simulink model "Suspension_model"  (R2023a)
settings: Solver=ode1  StartTime=0.0  StopTime=10  FixedStep=0.001  RelTol=1e-3
values from neighbouring files (symbols this model uses):
  A = [ 0 1 0 -1 ... (first row only)    [FitnessFunc.m]
  B = [0  0 ... (first row only)    [FitnessFunc.m]
  C = [ 1 0 0 0 ... (first row only)    [FitnessFunc.m]
  D = [0 0 ... (first row only)    [FitnessFunc.m]
  k = lqr(A, B(:, 2), Q, R)    [FitnessFunc.m]
undefined symbols (not defined in the file or in its folder): K
settings Model: Creator=ku53058  LastModifiedBy=sevva
settings SolverCC: AlgebraicLoopSolver=TrustRegion
settings DataIOCC: ReturnWorkspaceOutputs=off
settings OptimizationCC: LifeSpan=inf
settings DebuggingCC: UnconnectedInputMsg=warning  UnconnectedOutputMsg=warning  UnconnectedLineMsg=warning  ArithmeticOperatorsInVariantConditions=warning
settings ModelReferenceCC: EnableRefExpFcnMdlSchedulingChecks=on
settings SFSimCC: SimUseLocalCustomCode=off  CustomCodeUndefinedFunction=UseInterfaceOnly
settings RTWCC: RTWUseLocalCustomCode=off
settings CodeAppCC: StateflowObjectComments=on

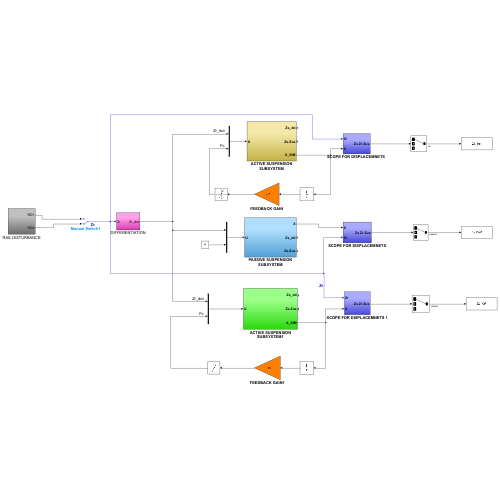
[thumbnail: Simulink's stored preview of the top-level diagram]
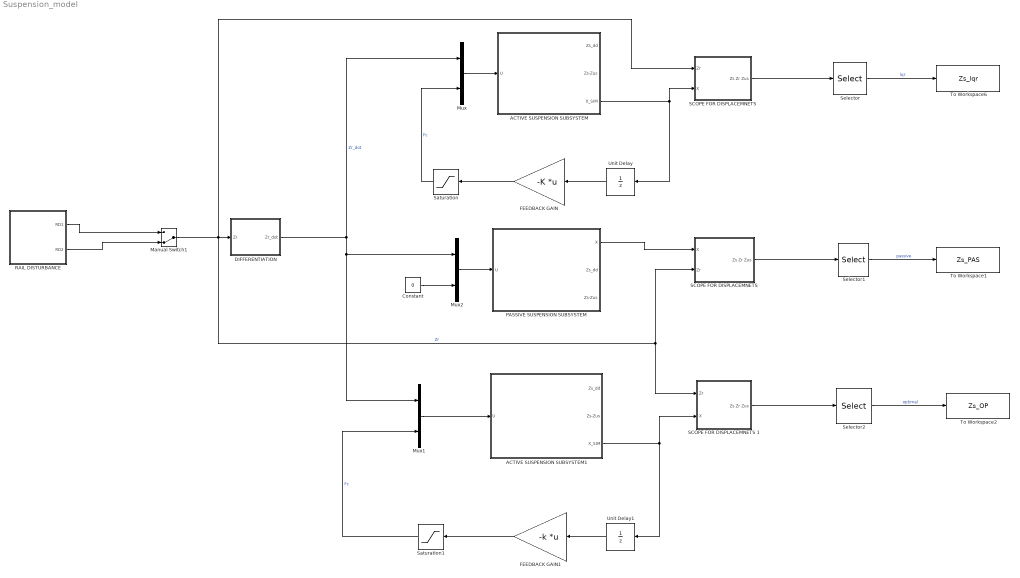
== system Suspension_model ==
  ACTIVE SUSPENSION SUBSYSTEM : Subsystem
  ACTIVE SUSPENSION SUBSYSTEM1 : Subsystem
  Constant : Constant  Value=0
  DIFFERENTIATION : Subsystem
  FEEDBACK GAIN : Gain  Gain=-K  Multiplication=Matrix(K*u)
  FEEDBACK GAIN1 : Gain  Gain=-k  Multiplication=Matrix(K*u)
  Manual Switch1 : ManualSwitch  CurrentSetting=0
  Mux : Mux  Inputs=2
  Mux1 : Mux  Inputs=2
  Mux2 : Mux  Inputs=2
  PASSIVE SUSPENSION SUBSYSTEM : Subsystem
  RAIL DISTURBANCE : Subsystem
  SCOPE FOR DISPLACEMNETS : Subsystem
  "SCOPE FOR DISPLACEMNETS " : Subsystem
  SCOPE FOR DISPLACEMNETS 1 : Subsystem
  Saturation : Saturate  UpperLimit=46730  LowerLimit=-46730
  Saturation1 : Saturate  UpperLimit=46730  LowerLimit=-46730
  Selector : Selector  InputPortWidth=3  IndexOptions=Index vector (dialog)  Indices=[1]  OutputSizes=1
  Selector1 : Selector  InputPortWidth=3  IndexOptions=Index vector (dialog)  Indices=[1]  OutputSizes=1
  Selector2 : Selector  InputPortWidth=3  IndexOptions=Index vector (dialog)  Indices=[1]  OutputSizes=1
  To Workspace1 : ToWorkspace  VariableName=Zs_PAS  SaveFormat=Timeseries  SampleTime=-1
  To Workspace2 : ToWorkspace  VariableName=Zs_OP  SaveFormat=Timeseries  SampleTime=-1
  To Workspace6 : ToWorkspace  VariableName=Zs_lqr  SaveFormat=Timeseries  SampleTime=-1
  Unit Delay : UnitDelay  SampleTime=-1  HasFrameUpgradeWarning=on
  Unit Delay1 : UnitDelay  SampleTime=-1  HasFrameUpgradeWarning=on
  wires:
  FEEDBACK GAIN/1 -> Saturation/1
  Constant/1 -> Mux2/2
  Unit Delay/1 -> FEEDBACK GAIN/1
  Saturation/1 -> Mux/2  "Fc"
  Mux/1 -> ACTIVE SUSPENSION SUBSYSTEM/1(U)
  ACTIVE SUSPENSION SUBSYSTEM/3(X_SIM) -> "SCOPE FOR DISPLACEMNETS "/2(X), Unit Delay/1
  "SCOPE FOR DISPLACEMNETS "/1(Zs Zr Zus) -> Selector/1
  Mux2/1 -> PASSIVE SUSPENSION SUBSYSTEM/1(U)
  PASSIVE SUSPENSION SUBSYSTEM/1(X) -> SCOPE FOR DISPLACEMNETS/1(X)
  SCOPE FOR DISPLACEMNETS/1(Zs Zr Zus) -> Selector1/1
  RAIL DISTURBANCE/1(RD1) -> Manual Switch1/1
  RAIL DISTURBANCE/2(RD2) -> Manual Switch1/2
  Selector/1 -> To Workspace6/1  "lqr"
  SCOPE FOR DISPLACEMNETS 1/1(Zs Zr Zus) -> Selector2/1
  Mux1/1 -> ACTIVE SUSPENSION SUBSYSTEM1/1(U)
  FEEDBACK GAIN1/1 -> Saturation1/1
  Unit Delay1/1 -> FEEDBACK GAIN1/1
  DIFFERENTIATION/1(Zr_dot) -> Mux/1, Mux1/1, Mux2/1  "Zr_dot"
  Saturation1/1 -> Mux1/2  "Fc"
  Manual Switch1/1 -> SCOPE FOR DISPLACEMNETS 1/1(Zr), SCOPE FOR DISPLACEMNETS/2(Zr), "SCOPE FOR DISPLACEMNETS "/1(Zr), DIFFERENTIATION/1(Zr)  "Zr"
  ACTIVE SUSPENSION SUBSYSTEM1/3(X_SIM) -> Unit Delay1/1, SCOPE FOR DISPLACEMNETS 1/2(X)
  Selector2/1 -> To Workspace2/1  "optimal"
  Selector1/1 -> To Workspace1/1  "passive"

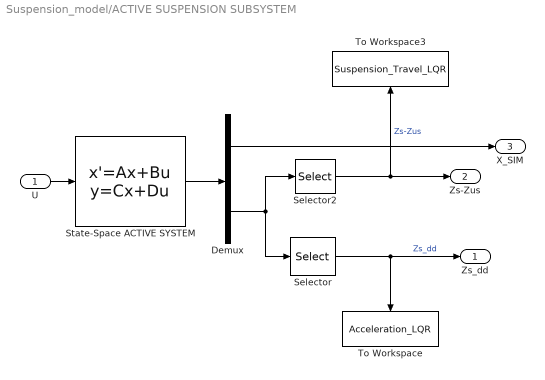
== system Suspension_model/ACTIVE SUSPENSION SUBSYSTEM ==
  U : Inport
  Demux : Demux  Outputs=[4 2]
  Selector : Selector  InputPortWidth=2  IndexOptions=Index vector (dialog)  Indices=[2]  OutputSizes=1
  Selector2 : Selector  InputPortWidth=2  IndexOptions=Index vector (dialog)  Indices=[1]  OutputSizes=1
  State-Space ACTIVE SYSTEM : StateSpace  A=A  B=B  C=cat(1,eye(4), C)  D=D  InitialCondition=0
  To Workspace : ToWorkspace  VariableName=Acceleration_LQR  SaveFormat=Timeseries  SampleTime=-1
  To Workspace3 : ToWorkspace  VariableName=Suspension_Travel_LQR  SaveFormat=Timeseries  SampleTime=-1
  Zs_dd : Outport
  Zs-Zus : Outport  Port=2
  X_SIM : Outport  Port=3
  wires:
  Demux/1 -> X_SIM/1
  State-Space ACTIVE SYSTEM/1 -> Demux/1
  Demux/2 -> Selector2/1, Selector/1
  Selector/1 -> Zs_dd/1, To Workspace/1  "Zs_dd"
  Selector2/1 -> Zs-Zus/1, To Workspace3/1  "Zs-Zus"
  U/1 -> State-Space ACTIVE SYSTEM/1

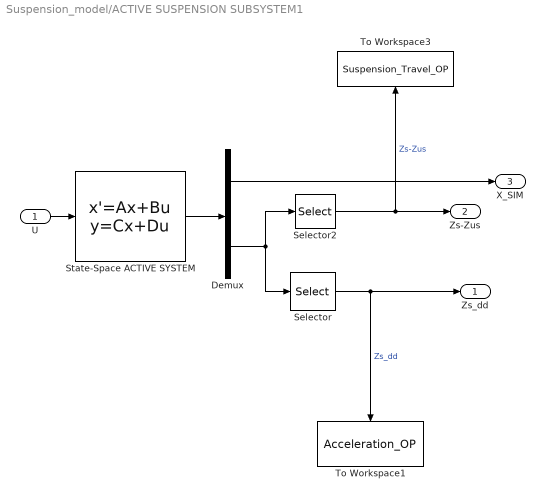
== system Suspension_model/ACTIVE SUSPENSION SUBSYSTEM1 ==
  U : Inport
  Demux : Demux  Outputs=[4 2]
  Selector : Selector  InputPortWidth=2  IndexOptions=Index vector (dialog)  Indices=[2]  OutputSizes=1
  Selector2 : Selector  InputPortWidth=2  IndexOptions=Index vector (dialog)  Indices=[1]  OutputSizes=1
  State-Space ACTIVE SYSTEM : StateSpace  A=A  B=B  C=cat(1,eye(4), C)  D=D  InitialCondition=0
  To Workspace1 : ToWorkspace  VariableName=Acceleration_OP  SaveFormat=Timeseries  SampleTime=-1
  To Workspace3 : ToWorkspace  VariableName=Suspension_Travel_OP  SaveFormat=Timeseries  SampleTime=-1
  Zs_dd : Outport
  Zs-Zus : Outport  Port=2
  X_SIM : Outport  Port=3
  wires:
  Demux/1 -> X_SIM/1
  State-Space ACTIVE SYSTEM/1 -> Demux/1
  Demux/2 -> Selector2/1, Selector/1
  Selector/1 -> To Workspace1/1, Zs_dd/1  "Zs_dd"
  Selector2/1 -> Zs-Zus/1, To Workspace3/1  "Zs-Zus"
  U/1 -> State-Space ACTIVE SYSTEM/1

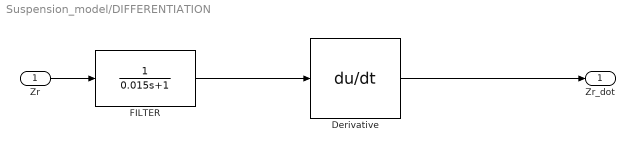
== system Suspension_model/DIFFERENTIATION ==
  Zr : Inport
  Derivative : Derivative
  FILTER : TransferFcn  Denominator=[0.015 1]
  Zr_dot : Outport
  wires:
  FILTER/1 -> Derivative/1
  Derivative/1 -> Zr_dot/1
  Zr/1 -> FILTER/1

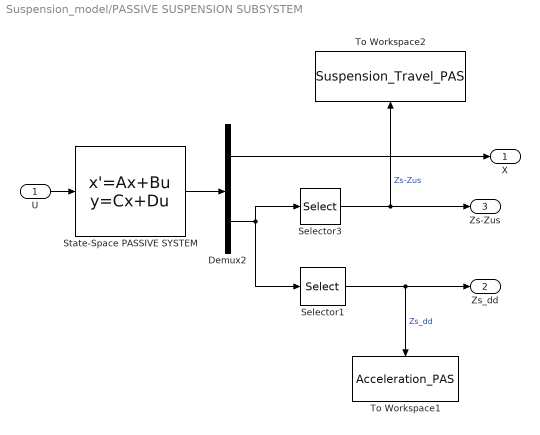
== system Suspension_model/PASSIVE SUSPENSION SUBSYSTEM ==
  U : Inport
  Demux2 : Demux  Outputs=[4 2]
  Selector1 : Selector  InputPortWidth=2  IndexOptions=Index vector (dialog)  Indices=[2]  OutputSizes=1
  Selector3 : Selector  InputPortWidth=2  IndexOptions=Index vector (dialog)  Indices=[1]  OutputSizes=1
  State-Space PASSIVE SYSTEM : StateSpace  A=A  B=B  C=cat(1,eye(4), C)  D=D  InitialCondition=0
  To Workspace1 : ToWorkspace  VariableName=Acceleration_PAS  SaveFormat=Timeseries  SampleTime=-1
  To Workspace2 : ToWorkspace  VariableName=Suspension_Travel_PAS  SaveFormat=Timeseries  SampleTime=-1
  X : Outport
  Zs_dd : Outport  Port=2
  Zs-Zus : Outport  Port=3
  wires:
  State-Space PASSIVE SYSTEM/1 -> Demux2/1
  Selector1/1 -> Zs_dd/1, To Workspace1/1  "Zs_dd"
  Demux2/2 -> Selector3/1, Selector1/1
  Selector3/1 -> Zs-Zus/1, To Workspace2/1  "Zs-Zus"
  U/1 -> State-Space PASSIVE SYSTEM/1
  Demux2/1 -> X/1

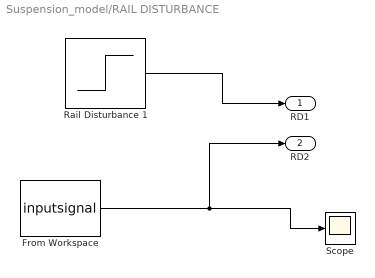
== system Suspension_model/RAIL DISTURBANCE ==
  From Workspace : FromWorkspace  VariableName=inputsignal
  Rail Disturbance 1 : Step  After=0.06  SampleTime=0
  Scope : Scope
  RD1 : Outport
  RD2 : Outport  Port=2
  wires:
  Rail Disturbance 1/1 -> RD1/1
  From Workspace/1 -> Scope/1, RD2/1

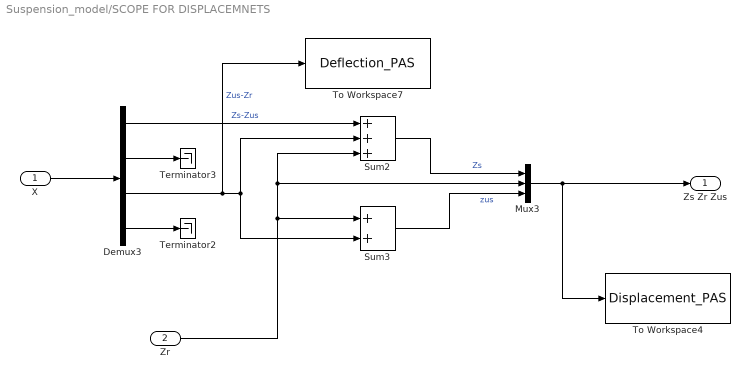
== system Suspension_model/SCOPE FOR DISPLACEMNETS ==
  X : Inport
  Zr : Inport  Port=2
  Demux3 : Demux
  Mux3 : Mux  Inputs=3
  Sum2 : Sum  Inputs=+++
  Sum3 : Sum
  Terminator2 : Terminator
  Terminator3 : Terminator
  To Workspace4 : ToWorkspace  VariableName=Displacement_PAS  SaveFormat=Timeseries  SampleTime=-1
  To Workspace7 : ToWorkspace  VariableName=Deflection_PAS  SaveFormat=Timeseries  SampleTime=-1
  Zs Zr Zus : Outport
  wires:
  Demux3/2 -> Terminator3/1
  Demux3/4 -> Terminator2/1
  Demux3/1 -> Sum2/1  "Zs-Zus"
  Demux3/3 -> To Workspace7/1, Sum3/2, Sum2/2  "Zus-Zr"
  Sum2/1 -> Mux3/1  "Zs"
  Sum3/1 -> Mux3/3  "zus"
  Mux3/1 -> Zs Zr Zus/1, To Workspace4/1
  Zr/1 -> Sum3/1, Mux3/2, Sum2/3
  X/1 -> Demux3/1

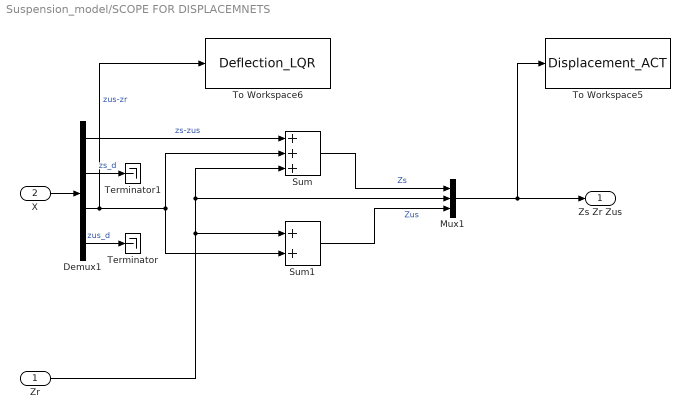
== system Suspension_model/SCOPE FOR DISPLACEMNETS  ==
  Zr : Inport
  X : Inport  Port=2
  Demux1 : Demux
  Mux1 : Mux  Inputs=3
  Sum : Sum  Inputs=+++
  Sum1 : Sum
  Terminator : Terminator
  Terminator1 : Terminator
  To Workspace5 : ToWorkspace  VariableName=Displacement_ACT  SaveFormat=Timeseries  SampleTime=-1
  To Workspace6 : ToWorkspace  VariableName=Deflection_LQR  SaveFormat=Timeseries  SampleTime=-1
  Zs Zr Zus : Outport
  wires:
  X/1 -> Demux1/1
  Demux1/2 -> Terminator1/1  "zs_d"
  Demux1/4 -> Terminator/1  "zus_d"
  Demux1/1 -> Sum/1  "zs-zus"
  Demux1/3 -> To Workspace6/1, Sum1/2, Sum/2  "zus-zr"
  Sum/1 -> Mux1/1  "Zs"
  Sum1/1 -> Mux1/3  "Zus"
  Mux1/1 -> Zs Zr Zus/1, To Workspace5/1
  Zr/1 -> Sum1/1, Mux1/2, Sum/3

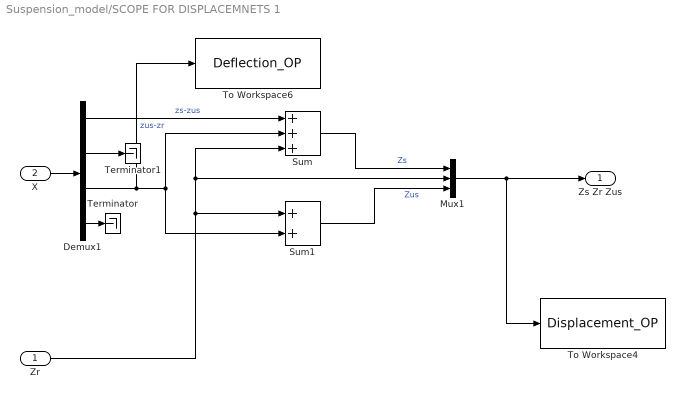
== system Suspension_model/SCOPE FOR DISPLACEMNETS 1 ==
  Zr : Inport
  X : Inport  Port=2
  Demux1 : Demux
  Mux1 : Mux  Inputs=3
  Sum : Sum  Inputs=+++
  Sum1 : Sum
  Terminator : Terminator
  Terminator1 : Terminator
  To Workspace4 : ToWorkspace  VariableName=Displacement_OP  SaveFormat=Timeseries  SampleTime=-1
  To Workspace6 : ToWorkspace  VariableName=Deflection_OP  SaveFormat=Timeseries  SampleTime=-1
  Zs Zr Zus : Outport
  wires:
  X/1 -> Demux1/1
  Demux1/2 -> Terminator1/1
  Demux1/4 -> Terminator/1
  Demux1/1 -> Sum/1  "zs-zus"
  Demux1/3 -> Sum1/2, Sum/2, To Workspace6/1  "zus-zr"
  Sum/1 -> Mux1/1  "Zs"
  Sum1/1 -> Mux1/3  "Zus"
  Mux1/1 -> To Workspace4/1, Zs Zr Zus/1
  Zr/1 -> Sum1/1, Mux1/2, Sum/3
